simulink model "d_tcsc"  (Simulink 5.1)
settings: Solver=ode45  StartTime=0.0  StopTime=10.0  RelTol=1e-3
libraries: fm_lib x6
settings Model: Creator=fmilano  LastModifiedBy=fmilano  ExtModeAutoUpdateStatusClock=off  SignalLoggingName=logsout  BooleanDataType=on  RTWOptions="-aEnforceIntegerDowncast=1 -aFoldNonRolledExpr=1 -aInlineInvariantSignals=1 -aInlineParameters=0 -aLocalBlockOutputs=1 -aRollThreshold=5 -aZeroInternalMemoryAtStartup=1 -aZeroExternalMemoryAtStartup=1 -aInitFltsAndDblsToZero=1 -aForceBlockIOInitOptimize=0 -aGenerateReport=0 -aGenCodeOnly=0 -aRTWVerbose=1 -aIncludeHyperlinkInReport=0 -aLaunchReport=0 -aGenerateTraceInfo=0  -aForceParamTrailComments=0 -aGenerateComments=1 -aIgnoreCustomStorageClasses=1 -aIncHierarchyInIds=0 -aMaxRTWIdLen=31 -aShowEliminatedStatements=0 -aIncDataTypeInIds=0 -aInsertBlockDesc=0 -aIgnoreTestpoints=0 -aSimulinkBlockComments=1 -aInlinedPrmAccess=\"Literals\"  -aSuppressErrorStatus=0 -aModelReferenceCompliant=1 -aParenthesesLevel=\"Nominal\" -aModelStepFunctionPrototypeControlCompliant=0 -aPortableWordSizes=0 -aParMdlRefBuildCompliant=1 -aSupportNonInlinedSFcns=1 -aSupportContinuousTime=1 -aSupportComplex=1 -aSupportNonFinite=1 -aSupportAbsoluteTime=1 -aMultiwordLength=2048 -aTargetPreCompLibLocation=\"\" -aTargetLibSuffix=\"\" -aTargetFunctionLibrary=\"ANSI_C\" -aTargetFcnLib=\"ansi_tfl_tmw.mat\" -aMultiInstanceERTCode=0 -aLogVarNameModifier=\"rt_\" -aERTFirstTimeCompliant=0 -aIsPILTarget=0 -aCombineOutputUpdateFcns=0 -aGenerateASAP2=0 -aGenerateClassInterface=0 -aGenerateTestInterfaces=0 -aGenerateSampleERTMain=0 -aGenerateFullHeader=1 -aUtilityFuncGeneration=\"Auto\" -aIncludeFileDelimiter=\"Auto\" -aIncludeMdlTerminateFcn=1 -aPurelyIntegerCode=0 -aAutosarCompliant=0 -aERTCustomFileBanners=0 -aRTWCAPIStates=0 -aRTWCAPIParams=0 -aRTWCAPISignals=0 -aMatFileLogging=1 -aCompOptLevelCompliant=0 -aCPPClassGenCompliant=0 -aExtModeIntrfLevel=\"Level1\" -aExtModeMexFile=\"ext_comm\" -aExtModeTransport=0 -aExtModeStaticAllocSize=1000000 -aExtModeTesting=0 -aExtModeStaticAlloc=0 -aExtMode=0 -aERTMultiwordLength=256 -aERTMultiwordTypeDef=\"System defined\"  -aGenerateTraceInfo=0 -aGenerateTraceInfo=0 -aGenerateTraceInfo=0 -aGenerateTraceInfo=0 -aPrefixModelToSubsysFcnNames=1"

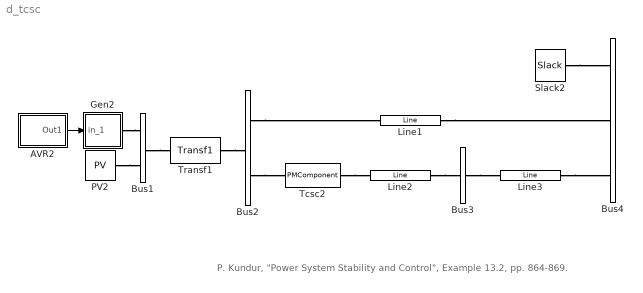
== system d_tcsc ==
  note: P. Kundur, "Power System Stability and Control", Example 13.2, pp. 864-869.
  AVR2 : Subsystem  Tag=PSATblock  Description=Controls  mask(Exc){p2q=3, p3q=7.00, p4q=-6.40, p5q=200, p6q=1, p7q=1, p8q=1.00, p9q=0.01, p10q=1.00, p11q=0.015, p12_13q=[0.0006  0.9], in=0}
      mask prompts: p2q "Automatic Voltage Regulator Type"; p3q "Maximum Regulator Voltage [p.u.]"; p4q "Minimum Regulator Voltage [p.u.]"; p5q "Regulator Gain [p.u./p.u.]"; p6q "Regulator Pole T2 [s]"; p7q "Regulator Zero T1 [s]"; p8q "Second Regulator Pole T3 [s]"; p9q "Allow signal V/V0 [0 for disabling signal]"; p10q "Time Constant of the Field Circuit Td [s]"; p11q "Time Delay of the Measurement System Tr [s]"; p12_13q "Coefficient of the Ceiling Function (A B)"; in "Number of input signals"
      mask help: This block defines an Automatic Voltage Regulator.
      mask init:
      | fm_inout
      | [x,y] = fm_draw('R');
      mask Help:
      | This block defines an Automatic Voltage Regulator.
      | There are three kind of regulators:
      | 
      | Type 1:
      | 
      |      IEEE Model 1
      | 
      | Type 2:
      | 
      |      IEEE Model 2
      | 
      | Type 3:
      | 
      |      IEEE Model 3
      mask StyleString: popup(1|2|3),edit,edit,edit,edit,edit,edit,edit,edit,edit,edit,popup(0|1|2|3)
      mask CallbackString: fm_block|||||||||||
      mask Display:
      | plot([-1.8 4.1 4.1 -1.8 -1.8],[-1.5 -1.5 1.5 1.5 -1.5])
      | color('red')
      | plot([-1.3 -0.5],[-1 1],[-0.5 0.3],[1 -1],[-0.9 -0.1],[0.0 0.0])
      | plot(2.8+1.3*x,2*y,1.5+[-1.3 -0.5],[1 -1],1.5+[-0.5 0.3],[-1 1])
  Bus1 : PMComponent  Tag=PSATblock  Description=Connection  PhysicalDomain=psatdomain  LeftPortType=p1  RightPortType=p1  LConnTagsString=__newl0|__newl1  RConnTagsString=__newr0  mask(Bus){in=2, out=1, p2q=24, p3_4q=[1.00   0.00], p5q=1, p6q=1}
      mask prompts: in "Number of inputs:"; out "Number of outputs:"; p2q "Voltage Rating [kV]"; p3_4q "Voltage initial guess [p.u.  rad]"; p5q "Area number"; p6q "Region number"
      mask help: Bus block.
      mask init:
      | fm_inout
      mask CallbackString: ||||fm_block|
      mask Display: plot([0 1 1 0 0],[0 0 1 1 0])
  Bus2 : PMComponent  Tag=PSATblock  Description=Connection  PhysicalDomain=psatdomain  LeftPortType=p1  RightPortType=p1  LConnTagsString=__newl0  RConnTagsString=__newr0|__newr1  mask(Bus){in=1, out=2, p2q=400, p3_4q=[1.00   0.00], p5q=1, p6q=1}
      mask prompts: in "Number of inputs:"; out "Number of outputs:"; p2q "Voltage Rating [kV]"; p3_4q "Voltage initial guess [p.u.  rad]"; p5q "Area number"; p6q "Region number"
      mask help: Bus block.
      mask init:
      | fm_inout
      mask CallbackString: ||||fm_block|
      mask Display: plot([0 1 1 0 0],[0 0 1 1 0])
  Bus3 : PMComponent  Tag=PSATblock  Description=Connection  PhysicalDomain=psatdomain  LeftPortType=p1  RightPortType=p1  LConnTagsString=__newl0  RConnTagsString=__newr0  mask(Bus){in=1, out=1, p2q=400, p3_4q=[1.00   0.00], p5q=1, p6q=1}
      mask prompts: in "Number of inputs:"; out "Number of outputs:"; p2q "Voltage Rating [kV]"; p3_4q "Voltage initial guess [p.u.  rad]"; p5q "Area number"; p6q "Region number"
      mask help: Bus block.
      mask init:
      | fm_inout
      mask CallbackString: ||||fm_block|
      mask Display: plot([0 1 1 0 0],[0 0 1 1 0])
  Bus4 : PMComponent  Tag=PSATblock  Description=Connection  PhysicalDomain=psatdomain  LeftPortType=p1  RightPortType=p1  LConnTagsString=__newl0|__newl1|__newl2  mask(Bus){in=3, out=0, p2q=400, p3_4q=[1.00   0.00], p5q=1, p6q=1}
      mask prompts: in "Number of inputs:"; out "Number of outputs:"; p2q "Voltage Rating [kV]"; p3_4q "Voltage initial guess [p.u.  rad]"; p5q "Area number"; p6q "Region number"
      mask help: Bus block.
      mask init:
      | fm_inout
      mask CallbackString: ||||fm_block|
      mask Display: plot([0 1 1 0 0],[0 0 1 1 0])
  Gen2 : Subsystem  Tag=PSATblock  Description=Machines  mask(Syn){p2_3_4q=[2220  24   60], p5q=6, p7_6q=[0.003  0.15], p8_9_10q=[1.81  0.30  0.23], p11_12q=[8.00  0.03], p13_14_15q=[1.76  0.65  0.25], p16_17q=[1.00  0.07], p18_19q=[7.00  0.00], p20_21q=[0.00  0.00], p22_23q=[1.00  1.00], p24q=0.00, p25_26q=[0.05  0.1], in=1}
      mask prompts: p2_3_4q "Power, voltage and frequency ratings [MVA, kV, Hz]"; p5q "Machine Dynamic Order"; p7_6q "resistance ra and leakage reactance xl [p.u. p.u.]"; p8_9_10q "d-axis reactances Xd, X'd X"d [p.u.,p.u.,p.u.]"; p11_12q "d-axis open circuit time constants T'd0 and T"d0 [s, s]"; p13_14_15q "q-axis reactances Xq, X'q, X"q [p.u.  p.u.  p.u.]"; p16_17q "q-axis open circuit time constants T'q0 and T"q0 [s s]"; p18_19q "Inertia (M = 2H) and Damping [s, p.u.]"; p20_21q "Speed and active power additional signals Kw & Kp [p.u., p.u.]"; p22_23q "Percentage of active and reactive powers at bus [p.u. p.u.]"; p24q "d-axis additional circuit leakage time constant Taa [s]"; p25_26q "Saturation coefficients S(1.0) and S(1.2)"; in "Number of input signals"
      mask help: This block defines a fourth order synchronous machine.
      mask init:
      | fm_inout
      | [x,y] = fm_draw('circle');
      | [xg,yg] = fm_draw('G');
      | [xs,ys] = fm_draw('sinus');
      mask StyleString: edit,popup(8|6|5.3|5.2|5.1|4|3|2),edit,edit,edit,edit,edit,edit,edit,edit,edit,edit,popup(0|1|2)
      mask CallbackString: |fm_block|||||||||||
      mask Display:
      | plot(x+1.4,y,0.12*xs+1,0.15*ys-0.6)
      | color('blue')
      | plot(1.4+0.45*xg,0.3+0.45*yg)
  Line1 : fm_lib/Power Flow/Line  Tag=PSATblock  Description=Power Flow  PhysicalDomain=psatdomain  SubClassName=unknown  LeftPortType=p1  RightPortType=p1  LConnTagsString=__newl0  RConnTagsString=__newr0  p3_4_5q="[2220  400  60]"  p6q=0  p8q=0.0  p9q=0.5  p10q=0.0  p13_14_15q="[0.0  0.0  0.0]"  p16q=on
  Line2 : fm_lib/Power Flow/Line  Tag=PSATblock  Description=Power Flow  PhysicalDomain=psatdomain  SubClassName=unknown  LeftPortType=p1  RightPortType=p1  LConnTagsString=__newl0  RConnTagsString=__newr0  p3_4_5q="[2220  400  60]"  p6q=0  p8q=0.01  p9q=0.8  p10q=0.0  p13_14_15q="[0.0  0.0  0.0]"  p16q=on
  Line3 : fm_lib/Power Flow/Line  Tag=PSATblock  Description=Power Flow  PhysicalDomain=psatdomain  SubClassName=unknown  LeftPortType=p1  RightPortType=p1  LConnTagsString=__newl0  RConnTagsString=__newr0  p3_4_5q="[2220  400  60]"  p6q=0  p8q=0.0  p9q=0.13  p10q=0.0  p13_14_15q="[0.0  0.0  0.0]"  p16q=on
  PV2 : fm_lib/Power Flow/PV  Tag=PSATblock  Description=Power Flow  PhysicalDomain=psatdomain  SubClassName=unknown  LeftPortType=p1  RightPortType=p1  RConnTagsString=__newr0  p2_3q="[2220  24]"  p4q=0.9  p5q=1.00  p6_7q="[0.8  -0.2]"  p8_9q="[1.1  0.9]"  p10q=1  p11q=on
  Slack2 : fm_lib/Power Flow/Slack  Tag=PSATblock  Description=Power Flow  PhysicalDomain=psatdomain  SubClassName=unknown  LeftPortType=p1  RightPortType=p1  RConnTagsString=__newr0  p2_3q="[2220  400]"  p4q=0.90081  p5q=0.00  p6_7q="[1.5  -1.5]"  p8_9q="[1.1  0.9]"  p10q=0.80  p11q=1  p12q=on  p13q=on
  Tcsc2 : PMComponent  Tag=PSATblock  Description=FACTS  PhysicalDomain=psatdomain  LeftPortType=p1  RightPortType=p1  LConnTagsString=__newl0  RConnTagsString=__newr0  mask(Tcsc){p5_6_7q=[2220 400  60], p2q=Alpha, p3q=constant_power_flow, p4q=constant_line_power, p8q=53.75, p9q=0.01, p10_11q=[3.1416  -3.1416], p12_13q=[5 1], p14_15q=[0.2  0.1], p16q=10, p17q=on}
      mask prompts: p5_6_7q "Power, Voltage and Frequency Ratings [MVA, kV, Hz]"; p2q "Model type:"; p3q "Operation mode:"; p4q "Scheduling strategy:"; p8q "Percentage of series compensation [%]"; p9q "Regulator time constant Tr [s]"; p10_11q "Alpha_max and Alpha_min [rad  rad]"; p12_13q "Proportional and Integral gains Kp and Ki"; p14_15q "XL and XC [p.u.  p.u.]"; p16q "Gain for stabilizing signal Kr [p.u./p.u.]"; p17q "Connected"
      mask help: This block describes a TCSC component.
      mask init:
      | [xi,yi] = fm_draw('ind');
      | [xc,yc] = fm_draw('cap');
      mask StyleString: edit,popup(Xc|Alpha),popup(constant_admittance|constant_power_flow),popup(constant_line_power|constant_angle),edit,edit,edit,edit,edit,edit,checkbox
      mask CallbackString: |fm_block|||||||||fm_block
      mask Display: plot([-1.6 -1.8 -1.8],[0.5 0.5 4],[0.2 0.2],[0.5 4],[-0.9 -0.9],[3 5],[0 0.2],[0.5 0.5],[-0.65 -0.85],[0.5 0.5],[-1.8 -0.9],[4 4],[0.2 -0.8],[4 4],[0.2 0.4],[1.9 1.9],[-1.8 -2],[1.9 1.9]), plot(-0.7+0.1*xc,4+yc,-1.15+0.175+0.125*yi,0.5+0.5*xi,-1.15-0.325+0.125*yi,0.5+0.5*xi,-1.15-0.075+0.125*yi,0.5+0.5*xi), color('magenta'), plot([-0.65 -0.65 0 0 -0.65],[-0.5 1.5 1.5 -0.5 -0.5],[-0.2 -0.45 -0.2 -0.2],[0 -0.5 -1 0],[-0.35 -0.35],[-0.7 -1.2],[-0.45 -0.45],[-1 0],[-0.45 -0.2 -0.45 -0.45],[1 1.5 2 1],[-0.2 -0.2],[2 1],[-0.3 -0.3],[1.7 2.2])
  Transf1 : fm_lib/Power Flow/Transf1  Tag=PSATblock  Description=Power Flow  PhysicalDomain=psatdomain  SubClassName=unknown  LeftPortType=p1  RightPortType=p1  LConnTagsString=__newl0  RConnTagsString=__newr0  p3_4_5q="[2220  24  60]"  p7q=24/400  p8q=0.0  p9q=0.15  p13_14_15q="[0.0  0.0  0.0]"  p16q=on
  wires:
  AVR2/1(Out1) -> Gen2/1(in_1)
  connections:
  Line3/RConn1 -- Bus4/LConn3
  Line1/RConn1 -- Bus4/LConn2
  Slack2/RConn1 -- Bus4/LConn1
  Bus3/RConn1 -- Line3/LConn1
  Line2/RConn1 -- Bus3/LConn1
  Bus2/RConn1 -- Line1/LConn1
  Transf1/RConn1 -- Bus2/LConn1
  Bus1/RConn1 -- Transf1/LConn1
  PV2/RConn1 -- Bus1/LConn2
  Gen2/RConn1 -- Bus1/LConn1
  Tcsc2/RConn1 -- Line2/LConn1
  Bus2/RConn2 -- Tcsc2/LConn1

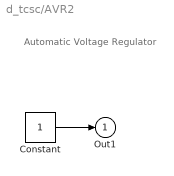
== system d_tcsc/AVR2 ==
  note: Automatic Voltage Regulator
  Constant : Constant  OutDataType=sfix(16)  OutScaling=2^0
  Out1 : Outport
  wires:
  Constant/1 -> Out1/1

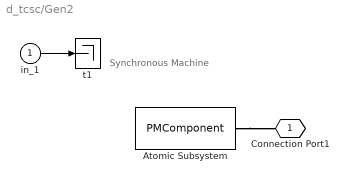
== system d_tcsc/Gen2 ==
  note: Synchronous Machine
  in_1 : Inport  OutDataType=sfix(16)  OutScaling=2^0
  Atomic Subsystem : PMComponent  PhysicalDomain=psatdomain  LeftPortType=p1  RightPortType=p1  RConnTagsString=__newr0
  t1 : Terminator
  Connection Port1 : PMIOPort  Tag=PMCPort  Orientation=left  Port=1  Side=Right
  wires:
  in_1/1 -> t1/1
  connections:
  Atomic Subsystem/RConn1 -- Connection Port1/RConn1
